simulink model "Consigne_cap"  (R2014a)
settings: Solver=ode3  StartTime=0.0  StopTime=inf  FixedStep=0.05  RelTol=1e-2
settings Model: Creator=Eric  LastModifiedBy=Andre
settings DataIOCC: SignalLoggingSaveFormat=ModelDataLogs
settings OptimizationCC: ExpressionDepthLimit=2147483647
settings DebuggingCC: UnderspecifiedInitializationDetection=Classic  FcnCallInpInsideContextMsg=EnableAllAsWarning  StateNameClashWarn=warning
settings GRTTargetCC: CombineOutputUpdateFcns=off  GRTInterface=on

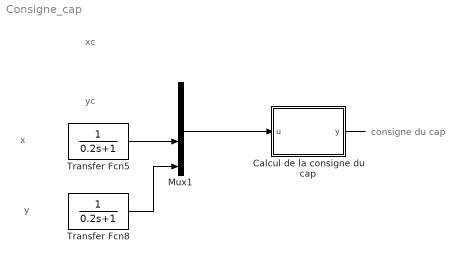
== system Consigne_cap ==
  note: consigne du cap
  note: y
  note: x
  note: yc
  note: xc
  Calcul de la consigne du cap : MATLAB Function  TreatAsAtomicUnit=on
  Mux1 : Mux
  Transfer Fcn5 : TransferFcn  Numerator=1  Denominator=[0.2 1]
  Transfer Fcn8 : TransferFcn  Numerator=1  Denominator=[0.2 1]
  wires:
  ? -> Mux1/1
  ? -> Mux1/2
  Mux1/1 -> Calcul de la consigne du cap/1(u)
  ? -> Transfer Fcn5/1
  Transfer Fcn5/1 -> Mux1/3
  ? -> Transfer Fcn8/1
  Transfer Fcn8/1 -> Mux1/4
  Calcul de la consigne du cap/1(y) -> ?

== matlab function Consigne_cap/Calcul de la consigne du cap ==
  data: u input; y output
function y = fcn(u)

persistent up;
if isempty(up)
    up=0;
end

w=unwrap([up atan2(u(2)-u(4),u(1)-u(3))]);

up=w(2);
y=up;
